simulink model "AMB_NL_2_simulation"  (R2021a)
settings: Solver=ode4  StartTime=0.0  StopTime=ttotal  FixedStep=dtsim  RelTol=1e-3
values from neighbouring files (symbols this model uses):
  a1_b0 = 2.13e13    (= 21300000000000)    [AMB_NL_1_vRTHS_m.m]
  a2 = 4.23e6    (= 4230000)    [AMB_NL_1_vRTHS_m.m]
  a3 = 3.3    [AMB_NL_1_vRTHS_m.m]
  adaptivegain = diag(10.^[8.4 6.2 2.1 0.8])    [AMB_NL_1_vRTHS_m.m]
  Ar = [zeros(3),eye(3);-M\Kmod -M\C]    [AMB_NL_1_vRTHS_m.m]
  asiv = 0.1    [AMB_NL_1_vRTHS_m.m]
  b1 = 425    [AMB_NL_1_vRTHS_m.m]
  b2 = 1e5    (= 100000)    [AMB_NL_1_vRTHS_m.m]
  Br = [zeros(3,2);-ones(3,1),-M\G2]    [AMB_NL_1_vRTHS_m.m]
  ce = 114.6    [AMB_NL_1_vRTHS_m.m]
  Cr = [eye(6)]    [AMB_NL_1_vRTHS_m.m]
  Derivadas = [u;dudt;dudt2;dudt3]    [AMB_NL_1_vRTHS_m.m]
  Dr = [zeros(6,2)]    [AMB_NL_1_vRTHS_m.m]
  dtsim = 1/fs    (= 0.000244140625)    [AMB_NL_1_vRTHS_m.m]
  dudt2 = [1 -2 1 0]/dtsim^2    [AMB_NL_1_vRTHS_m.m]
  gain = 1    [AMB_NL_1_vRTHS_m.m]
  ke = 1.19*10^6    (= 1190000)    [AMB_NL_1_vRTHS_m.m]
  khard = 6e9*0    (= 0)    [AMB_NL_1_vRTHS_m.m]
  max_amb = [amb0max,amb1max,amb2max,amb3max]    [AMB_NL_1_vRTHS_m.m]
  me = 29.1    [AMB_NL_1_vRTHS_m.m]
  min_amb = [amb0min,amb1min,amb2min,amb3min]    [AMB_NL_1_vRTHS_m.m]
  n1siv = 0.1    [AMB_NL_1_vRTHS_m.m]
  n2siv = 1-n1siv    (= 0.9)    [AMB_NL_1_vRTHS_m.m]
  nsiv = 2.5    [AMB_NL_1_vRTHS_m.m]
  rms_noise_desp = 6.25e-14    [AMB_NL_1_vRTHS_m.m]
  rms_noise_F = 1.16e-3    (= 0.00116)    [AMB_NL_1_vRTHS_m.m]
  sat_limit_lower = -3.8    [AMB_NL_1_vRTHS_m.m]
  sat_limit_upper = +3.8    (= 3.8)    [AMB_NL_1_vRTHS_m.m]
  ssAe = [0,1;-asiv*ke/me,-ce/me]    [AMB_NL_1_vRTHS_m.m]
  ssAn = [zeros(3),eye(3);-Mn\Kn,-Mn\Cn]    [AMB_NL_1_vRTHS_m.m]
  ssBe = [0,0;1/me,-1/me]    [AMB_NL_1_vRTHS_m.m]
  ssBn = [zeros(3,2);-Mn\M*G1,-Mn\G2]    [AMB_NL_1_vRTHS_m.m]
  ssCe = [1,0;0,1;asiv*ke,0]    [AMB_NL_1_vRTHS_m.m]
  ssCn = [eye(3),zeros(3)]    [AMB_NL_1_vRTHS_m.m]
  ssDe = [0,0;0,0;0,1]    [AMB_NL_1_vRTHS_m.m]
  ssDn = zeros(3,2)    [AMB_NL_1_vRTHS_m.m]
  stiffdeg = 0.02*0    (= 0)    [AMB_NL_1_vRTHS_m.m]
  strdeg = 0.005*0    (= 0)    [AMB_NL_1_vRTHS_m.m]
  xy = 1/1000    (= 0.001)    [AMB_NL_1_vRTHS_m.m]
undefined symbols (not defined in the file or in its folder): denfilter, DiscIntNeverNeededParam, numfilter
libraries: simulink x2
settings Model: Creator=cristobal  LastModifiedBy=MSI
settings SolverCC: AlgebraicLoopSolver=TrustRegion
settings DataIOCC: ReturnWorkspaceOutputs=off
settings DebuggingCC: SFMachineParentedDataDiag=warning  ArithmeticOperatorsInVariantConditions=warning
settings SFSimCC: SimUseLocalCustomCode=off  CustomCodeUndefinedFunction=UseInterfaceOnly
settings RTWCC: RTWUseLocalCustomCode=off
settings CodeAppCC: StateflowObjectComments=on

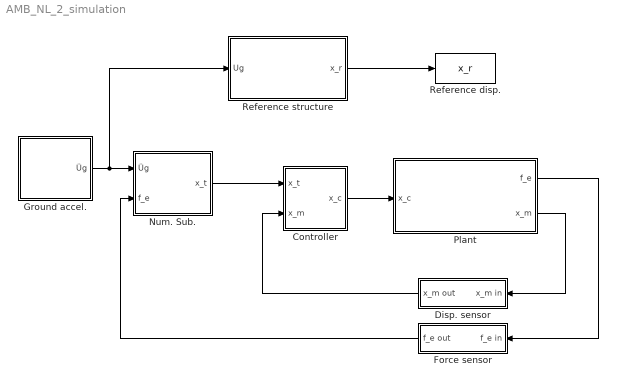
== system AMB_NL_2_simulation ==
  Controller : Subsystem
  Disp. sensor : Subsystem
  Force sensor : Subsystem
  Ground accel. : Subsystem
  Num. Sub. : Subsystem
  Plant : Subsystem
  Reference disp. : ToWorkspace  VariableName=x_r  SaveFormat=Timeseries  SampleTime=-1
  Reference structure : Subsystem
  wires:
  Num. Sub./1(x_t) -> Controller/1(x_t)
  Controller/1(x_c) -> Plant/1(x_c)
  Plant/1(f_e) -> Force sensor/1(f_e in)
  Plant/2(x_m) -> Disp. sensor/1(x_m in)
  Ground accel./1(Üg) -> Num. Sub./1(Üg), Reference structure/1(Ug)
  Reference structure/1(x_r) -> Reference disp./1
  Disp. sensor/1(x_m out) -> Controller/2(x_m)
  Force sensor/1(f_e out) -> Num. Sub./2(f_e)

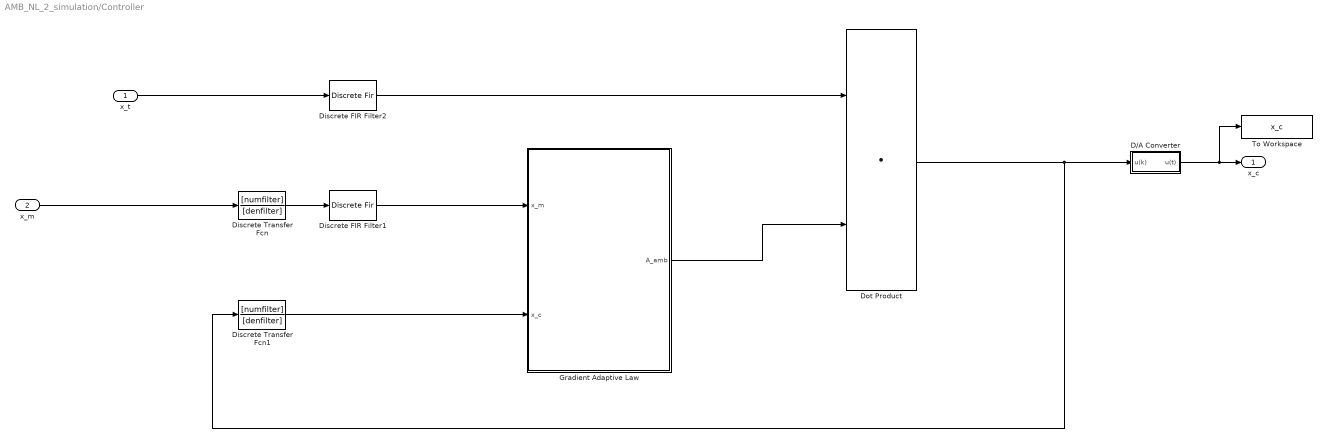
== system AMB_NL_2_simulation/Controller ==
  x_t : Inport
  x_m : Inport  Port=2
  D/A Converter : Subsystem
  Discrete Transfer Fcn : DiscreteTransferFcn  Numerator=[numfilter]  Denominator=[denfilter]
  Discrete Transfer Fcn1 : DiscreteTransferFcn  Numerator=[numfilter]  Denominator=[denfilter]
  Discrete FIR Filter1 : DiscreteFir  Coefficients=Derivadas
  Discrete FIR Filter2 : DiscreteFir  Coefficients=Derivadas
  Dot Product : DotProduct  InputSameDT=on  OutDataTypeStr=Inherit: Inherit via internal rule
  Gradient Adaptive Law : Subsystem
  To Workspace : ToWorkspace  VariableName=x_c  SaveFormat=Timeseries  SampleTime=-1
  x_c : Outport  VectorParamsAs1DForOutWhenUnconnected=off
  wires:
  Gradient Adaptive Law/1(A_amb) -> Dot Product/2
  Discrete FIR Filter1/1 -> Gradient Adaptive Law/1(x_m)
  Discrete Transfer Fcn1/1 -> Gradient Adaptive Law/2(x_c)
  x_m/1 -> Discrete Transfer Fcn/1
  Discrete Transfer Fcn/1 -> Discrete FIR Filter1/1
  x_t/1 -> Discrete FIR Filter2/1
  Dot Product/1 -> D/A Converter/1(u(k)), Discrete Transfer Fcn1/1
  Discrete FIR Filter2/1 -> Dot Product/1
  D/A Converter/1(u(t)) -> To Workspace/1, x_c/1

== system AMB_NL_2_simulation/Disp. sensor ==
  x_m in : Inport
  Band-Limited White Noise : simulink/Sources/Band-Limited White Noise  Cov=[rms_noise_desp]  Ts=dtsim  seed=ceil(rand(1)*10000)
  Sum : Sum  Inputs=|++
  To Workspace : ToWorkspace  VariableName=x_m  SaveFormat=Timeseries  SampleTime=-1
  To Workspace1 : ToWorkspace  VariableName=noise_desp  SaveFormat=Timeseries  SampleTime=-1
  x_m out : Outport  VectorParamsAs1DForOutWhenUnconnected=off
  wires:
  Band-Limited White Noise/1 -> To Workspace1/1, Sum/2
  Sum/1 -> x_m out/1, To Workspace/1
  x_m in/1 -> Sum/1

== system AMB_NL_2_simulation/Force sensor ==
  f_e in : Inport
  Band-Limited White Noise : simulink/Sources/Band-Limited White Noise  Cov=[rms_noise_F]  Ts=dtsim  seed=ceil(rand(1)*100)
  Sum : Sum  Inputs=|++
  To Workspace : ToWorkspace  VariableName=F_m  SaveFormat=Timeseries  SampleTime=-1
  f_e out : Outport  VectorParamsAs1DForOutWhenUnconnected=off
  wires:
  f_e in/1 -> Sum/1
  Sum/1 -> To Workspace/1, f_e out/1
  Band-Limited White Noise/1 -> Sum/2

== system AMB_NL_2_simulation/Ground accel. ==
  From Workspace1 : FromWorkspace  VariableName=Ug  OutputAfterFinalValue=Setting to zero
  To Workspace : ToWorkspace  VariableName=Ugs  SaveFormat=Timeseries  SampleTime=-1
  Üg : Outport  VectorParamsAs1DForOutWhenUnconnected=off
  wires:
  From Workspace1/1 -> To Workspace/1, Üg/1

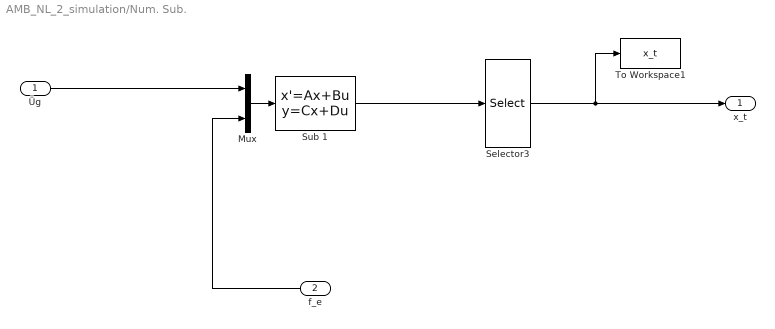
== system AMB_NL_2_simulation/Num. Sub. ==
  Üg : Inport
  f_e : Inport  Port=2
  Mux : Mux  Inputs=2
  Selector3 : Selector  InputPortWidth=3  IndexOptions=Index vector (dialog)  Indices=[1]  OutputSizes=1
  Sub 1 : StateSpace  A=ssAn  B=ssBn  C=ssCn  D=ssDn  InitialCondition=0
  To Workspace1 : ToWorkspace  VariableName=x_t  SaveFormat=Timeseries  SampleTime=-1
  x_t : Outport  VectorParamsAs1DForOutWhenUnconnected=off
  wires:
  Mux/1 -> Sub 1/1
  Selector3/1 -> x_t/1, To Workspace1/1
  Üg/1 -> Mux/1
  Sub 1/1 -> Selector3/1
  f_e/1 -> Mux/2

== system AMB_NL_2_simulation/Plant ==
  x_c : Inport
  Actuator : Subsystem
  Experimental Sub : Subsystem
  f_e : Outport  VectorParamsAs1DForOutWhenUnconnected=off
  x_m : Outport  Port=2  VectorParamsAs1DForOutWhenUnconnected=off
  wires:
  x_c/1 -> Actuator/1(x_c)
  Experimental Sub/2(x_m) -> x_m/1, Actuator/2(x_m)
  Experimental Sub/3(x_m s) -> Actuator/3(x_m s)
  Actuator/1(F) -> Experimental Sub/1(F)
  Experimental Sub/1(F2) -> f_e/1

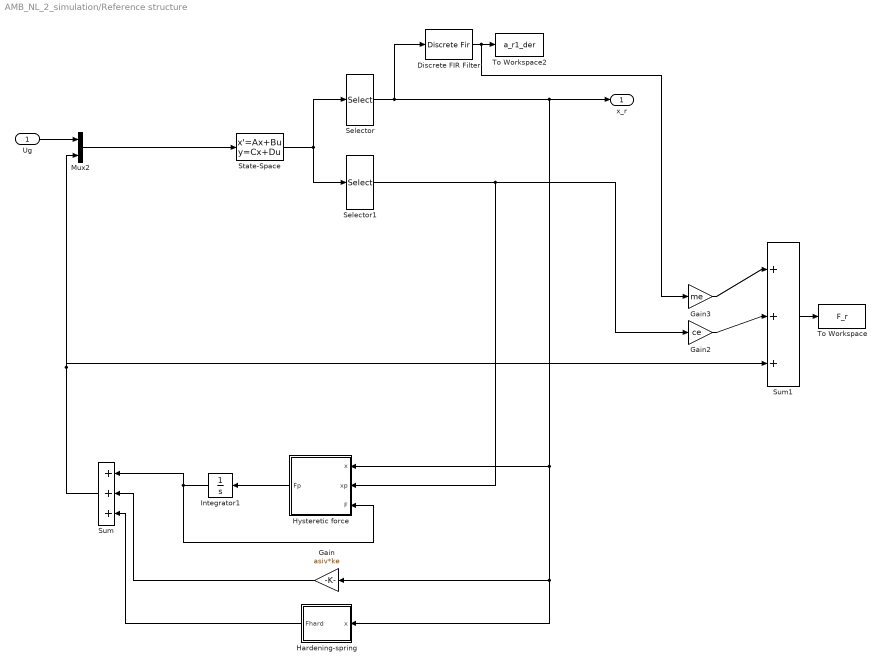
== system AMB_NL_2_simulation/Reference structure ==
  Ug : Inport
  Discrete FIR Filter : DiscreteFir  Coefficients=[dudt2]
  Gain : Gain  Gain=asiv*ke
  Gain2 : Gain  Gain=ce
  Gain3 : Gain  Gain=me
  Hardening-spring : Subsystem
  Hysteretic force : Subsystem
  Integrator1 : Integrator
  Mux2 : Mux  Inputs=2
  Selector : Selector  InputPortWidth=6  IndexOptions=Index vector (dialog)  Indices=[1]  OutputSizes=1
  Selector1 : Selector  InputPortWidth=6  IndexOptions=Index vector (dialog)  Indices=[4]  OutputSizes=1
  State-Space : StateSpace  A=Ar  B=Br  C=Cr  D=Dr  InitialCondition=0
  Sum : Sum  Inputs=|+++
  Sum1 : Sum  Inputs=|+++
  To Workspace : ToWorkspace  VariableName=F_r  SaveFormat=Timeseries  SampleTime=-1
  To Workspace2 : ToWorkspace  VariableName=a_r1_der  SaveFormat=Timeseries  SampleTime=-1
  x_r : Outport  VectorParamsAs1DForOutWhenUnconnected=off
  wires:
  State-Space/1 -> Selector1/1, Selector/1
  Selector/1 -> Discrete FIR Filter/1, Hardening-spring/1(x), Gain/1, Hysteretic force/1(x), x_r/1
  Selector1/1 -> Hysteretic force/2(xp), Gain2/1
  Mux2/1 -> State-Space/1
  Ug/1 -> Mux2/1
  Integrator1/1 -> Hysteretic force/3(F), Sum/1
  Gain/1 -> Sum/2
  Sum1/1 -> To Workspace/1
  Discrete FIR Filter/1 -> Gain3/1, To Workspace2/1
  Gain2/1 -> Sum1/2
  Gain3/1 -> Sum1/1
  Hysteretic force/1(Fp) -> Integrator1/1
  Sum/1 -> Mux2/2, Sum1/3
  Hardening-spring/1(Fhard) -> Sum/3

== system AMB_NL_2_simulation/Controller/D//A Converter ==
  u(k) : Inport
  Quantizer : Quantizer  QuantizationInterval=quantize_int
  Saturation : Saturate  UpperLimit=sat_limit_upper  LowerLimit=sat_limit_lower
  u(t) : Outport  VectorParamsAs1DForOutWhenUnconnected=off
  wires:
  Saturation/1 -> u(t)/1
  Quantizer/1 -> Saturation/1
  u(k)/1 -> Quantizer/1

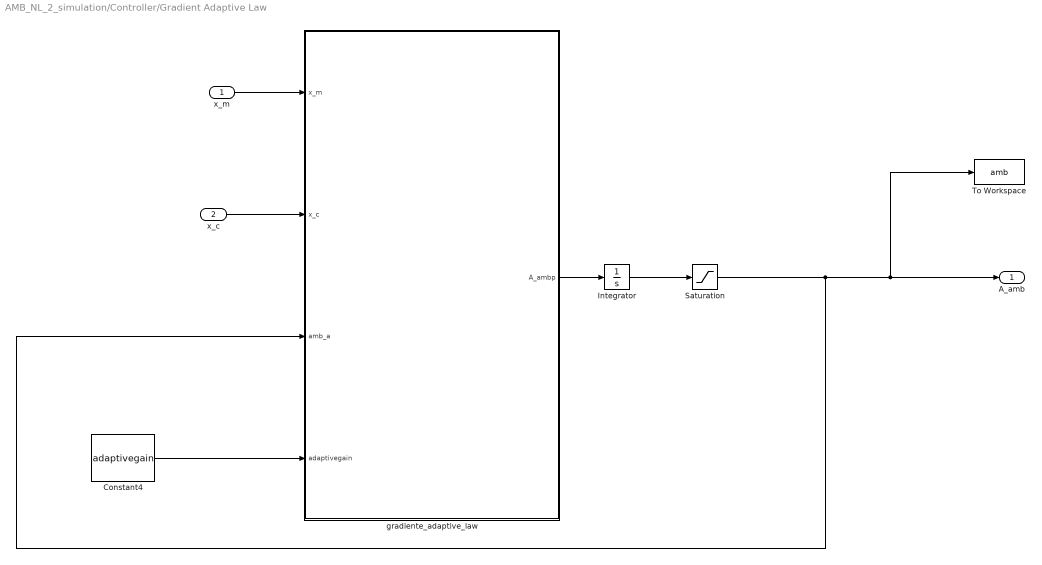
== system AMB_NL_2_simulation/Controller/Gradient Adaptive Law ==
  x_m : Inport
  x_c : Inport  Port=2
  Constant4 : Constant  Value=adaptivegain
  Integrator : Integrator  InitialCondition=A_amb_i'
  Saturation : Saturate  UpperLimit=[max_amb]  LowerLimit=min_amb
  To Workspace : ToWorkspace  VariableName=amb  SaveFormat=Timeseries  SampleTime=-1
  gradiente_adaptive_law : MATLAB Function  TreatAsAtomicUnit=on
  A_amb : Outport  VectorParamsAs1DForOutWhenUnconnected=off
  wires:
  Saturation/1 -> gradiente_adaptive_law/3(amb_a), To Workspace/1, A_amb/1
  Integrator/1 -> Saturation/1
  x_c/1 -> gradiente_adaptive_law/2(x_c)
  Constant4/1 -> gradiente_adaptive_law/4(adaptivegain)
  gradiente_adaptive_law/1(A_ambp) -> Integrator/1
  x_m/1 -> gradiente_adaptive_law/1(x_m)

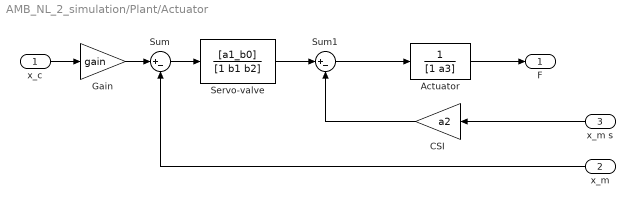
== system AMB_NL_2_simulation/Plant/Actuator ==
  x_c : Inport
  x_m : Inport  Port=2
  x_m s : Inport  Port=3
  Actuator : TransferFcn  Denominator=[1 a3]
  CSI : Gain  Gain=a2
  Gain : Gain  Gain=gain
  Servo-valve : TransferFcn  Numerator=[a1_b0]  Denominator=[1 b1 b2]
  Sum : Sum  Inputs=|+-
  Sum1 : Sum  Inputs=|+-
  F : Outport  VectorParamsAs1DForOutWhenUnconnected=off
  wires:
  CSI/1 -> Sum1/2
  Actuator/1 -> F/1
  Sum1/1 -> Actuator/1
  Sum/1 -> Servo-valve/1
  Servo-valve/1 -> Sum1/1
  x_c/1 -> Gain/1
  Gain/1 -> Sum/1
  x_m/1 -> Sum/2
  x_m s/1 -> CSI/1

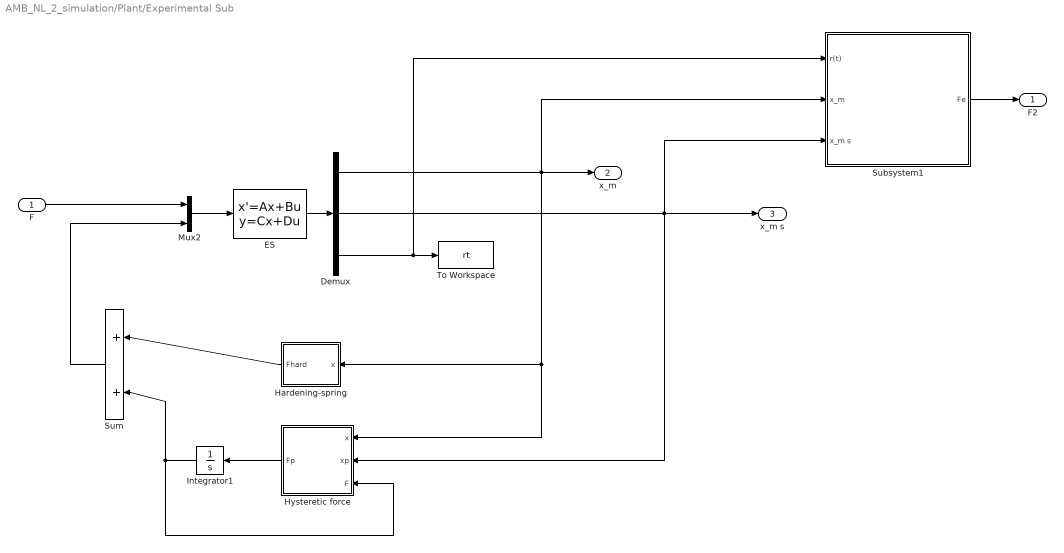
== system AMB_NL_2_simulation/Plant/Experimental Sub ==
  F : Inport
  Demux : Demux  Outputs=3
  ES : StateSpace  A=ssAe  B=ssBe  C=ssCe  D=ssDe  InitialCondition=0
  Hardening-spring : Subsystem
  Hysteretic force : Subsystem
  Integrator1 : Integrator
  Mux2 : Mux  Inputs=2
  Subsystem1 : Subsystem
  Sum : Sum  Inputs=|++
  To Workspace : ToWorkspace  VariableName=rt  SaveFormat=Timeseries  SampleTime=-1
  F2 : Outport  VectorParamsAs1DForOutWhenUnconnected=off
  x_m : Outport  Port=2  VectorParamsAs1DForOutWhenUnconnected=off
  x_m s : Outport  Port=3  VectorParamsAs1DForOutWhenUnconnected=off
  wires:
  ES/1 -> Demux/1
  F/1 -> Mux2/1
  Mux2/1 -> ES/1
  Demux/3 -> Subsystem1/1(r(t)), To Workspace/1
  Hysteretic force/1(Fp) -> Integrator1/1
  Demux/2 -> Hysteretic force/2(xp), Subsystem1/3(x_m s), x_m s/1
  Subsystem1/1(Fe) -> F2/1
  Demux/1 -> x_m/1, Hysteretic force/1(x), Hardening-spring/1(x), Subsystem1/2(x_m)
  Integrator1/1 -> Sum/2, Hysteretic force/3(F)
  Sum/1 -> Mux2/2
  Hardening-spring/1(Fhard) -> Sum/1

== system AMB_NL_2_simulation/Reference structure/Hardening-spring ==
  x : Inport
  Constant1 : Constant  Value=khard
  MATLAB Function : MATLAB Function  TreatAsAtomicUnit=on
  Unit Delay : UnitDelay  SampleTime=-1  HasFrameUpgradeWarning=on
  Fhard : Outport  VectorParamsAs1DForOutWhenUnconnected=off
  wires:
  x/1 -> Unit Delay/1
  Constant1/1 -> MATLAB Function/2(khard)
  MATLAB Function/1(Fhard) -> Fhard/1
  Unit Delay/1 -> MATLAB Function/1(x)

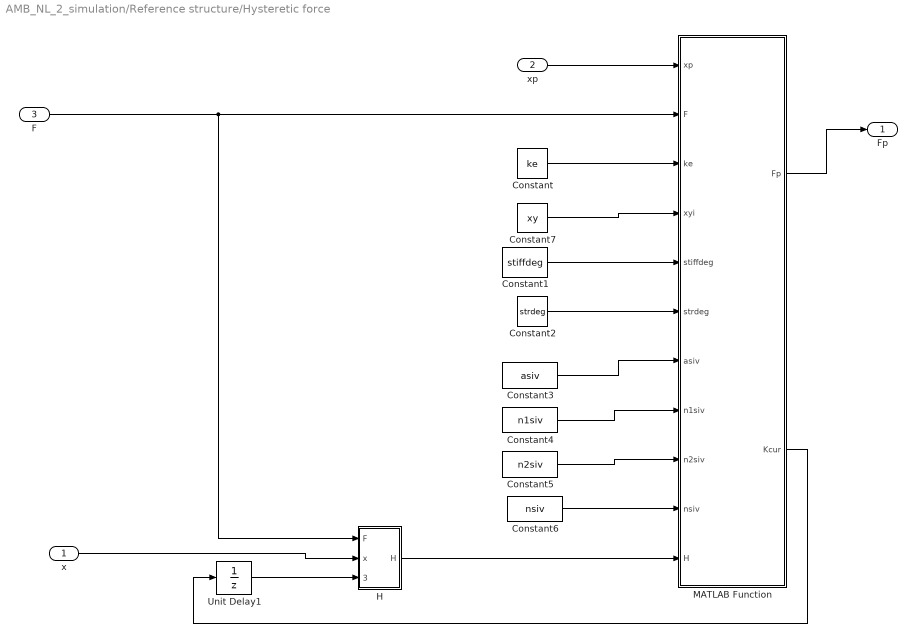
== system AMB_NL_2_simulation/Reference structure/Hysteretic force ==
  x : Inport
  xp : Inport  Port=2
  F : Inport  Port=3
  Constant : Constant  Value=ke
  Constant1 : Constant  Value=stiffdeg
  Constant2 : Constant  Value=strdeg
  Constant3 : Constant  Value=asiv
  Constant4 : Constant  Value=n1siv
  Constant5 : Constant  Value=n2siv
  Constant6 : Constant  Value=nsiv
  Constant7 : Constant  Value=xy
  H : Subsystem
  MATLAB Function : MATLAB Function  TreatAsAtomicUnit=on
  Unit Delay1 : UnitDelay  InitialCondition=ke  SampleTime=-1  HasFrameUpgradeWarning=on
  Fp : Outport  VectorParamsAs1DForOutWhenUnconnected=off
  wires:
  MATLAB Function/1(Fp) -> Fp/1
  MATLAB Function/2(Kcur) -> Unit Delay1/1
  x/1 -> H/2(x)
  xp/1 -> MATLAB Function/1(xp)
  Constant/1 -> MATLAB Function/3(ke)
  Constant7/1 -> MATLAB Function/4(xyi)
  Constant1/1 -> MATLAB Function/5(stiffdeg)
  Constant2/1 -> MATLAB Function/6(strdeg)
  Constant3/1 -> MATLAB Function/7(asiv)
  Constant4/1 -> MATLAB Function/8(n1siv)
  Constant5/1 -> MATLAB Function/9(n2siv)
  Constant6/1 -> MATLAB Function/10(nsiv)
  H/1(H) -> MATLAB Function/11(H)
  Unit Delay1/1 -> H/3("Kcur ")
  F/1 -> H/1(F), MATLAB Function/2(F)

== system AMB_NL_2_simulation/Plant/Experimental Sub/Hardening-spring ==
  x : Inport
  Constant1 : Constant  Value=khard
  MATLAB Function : MATLAB Function  TreatAsAtomicUnit=on
  Unit Delay : UnitDelay  SampleTime=-1  HasFrameUpgradeWarning=on
  Fhard : Outport  VectorParamsAs1DForOutWhenUnconnected=off
  wires:
  x/1 -> Unit Delay/1
  Constant1/1 -> MATLAB Function/2(khard)
  MATLAB Function/1(Fhard) -> Fhard/1
  Unit Delay/1 -> MATLAB Function/1(x)

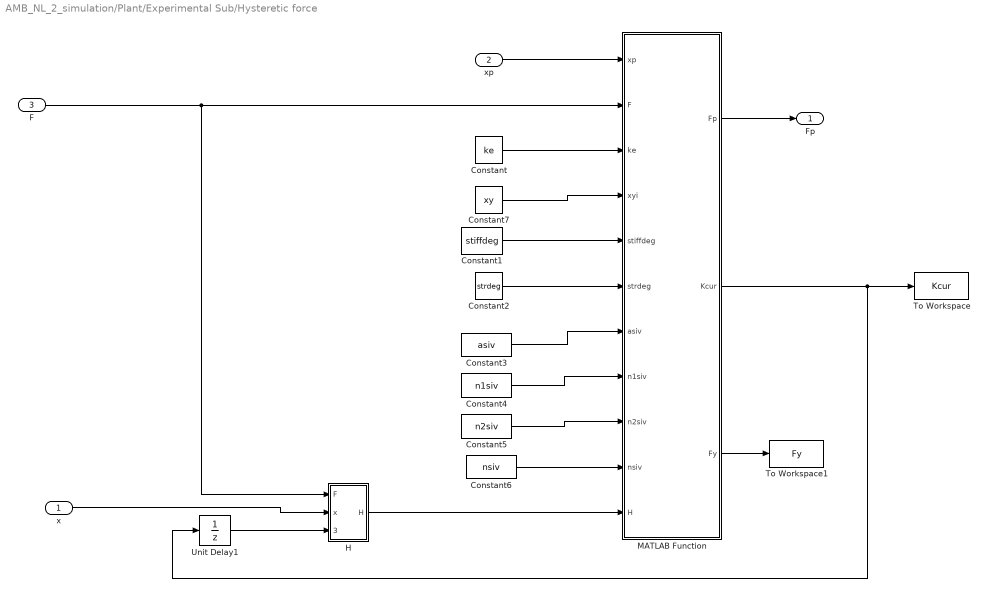
== system AMB_NL_2_simulation/Plant/Experimental Sub/Hysteretic force ==
  x : Inport
  xp : Inport  Port=2
  F : Inport  Port=3
  Constant : Constant  Value=ke
  Constant1 : Constant  Value=stiffdeg
  Constant2 : Constant  Value=strdeg
  Constant3 : Constant  Value=asiv
  Constant4 : Constant  Value=n1siv
  Constant5 : Constant  Value=n2siv
  Constant6 : Constant  Value=nsiv
  Constant7 : Constant  Value=xy
  H : Subsystem
  MATLAB Function : MATLAB Function  TreatAsAtomicUnit=on
  To Workspace : ToWorkspace  VariableName=Kcur  SaveFormat=Timeseries  SampleTime=-1
  To Workspace1 : ToWorkspace  VariableName=Fy  SaveFormat=Timeseries  SampleTime=-1
  Unit Delay1 : UnitDelay  InitialCondition=ke  SampleTime=-1  HasFrameUpgradeWarning=on
  Fp : Outport  VectorParamsAs1DForOutWhenUnconnected=off
  wires:
  MATLAB Function/1(Fp) -> Fp/1
  MATLAB Function/2(Kcur) -> Unit Delay1/1, To Workspace/1
  x/1 -> H/2(x)
  xp/1 -> MATLAB Function/1(xp)
  Constant/1 -> MATLAB Function/3(ke)
  Constant7/1 -> MATLAB Function/4(xyi)
  Constant1/1 -> MATLAB Function/5(stiffdeg)
  Constant2/1 -> MATLAB Function/6(strdeg)
  Constant3/1 -> MATLAB Function/7(asiv)
  Constant4/1 -> MATLAB Function/8(n1siv)
  Constant5/1 -> MATLAB Function/9(n2siv)
  Constant6/1 -> MATLAB Function/10(nsiv)
  H/1(H) -> MATLAB Function/11(H)
  Unit Delay1/1 -> H/3("Kcur ")
  F/1 -> H/1(F), MATLAB Function/2(F)
  MATLAB Function/3(Fy) -> To Workspace1/1

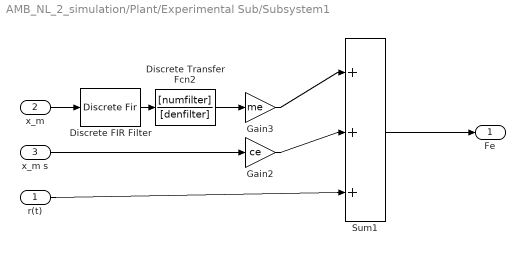
== system AMB_NL_2_simulation/Plant/Experimental Sub/Subsystem1 ==
  r(t) : Inport
  x_m : Inport  Port=2
  x_m s : Inport  Port=3
  Discrete Transfer Fcn2 : DiscreteTransferFcn  Numerator=[numfilter]  Denominator=[denfilter]
  Discrete FIR Filter : DiscreteFir  Coefficients=[dudt2]
  Gain2 : Gain  Gain=ce
  Gain3 : Gain  Gain=me
  Sum1 : Sum  Inputs=|+++
  Fe : Outport  VectorParamsAs1DForOutWhenUnconnected=off
  wires:
  Sum1/1 -> Fe/1
  Discrete FIR Filter/1 -> Discrete Transfer Fcn2/1
  Discrete Transfer Fcn2/1 -> Gain3/1
  Gain3/1 -> Sum1/1
  Gain2/1 -> Sum1/2
  r(t)/1 -> Sum1/3
  x_m s/1 -> Gain2/1
  x_m/1 -> Discrete FIR Filter/1

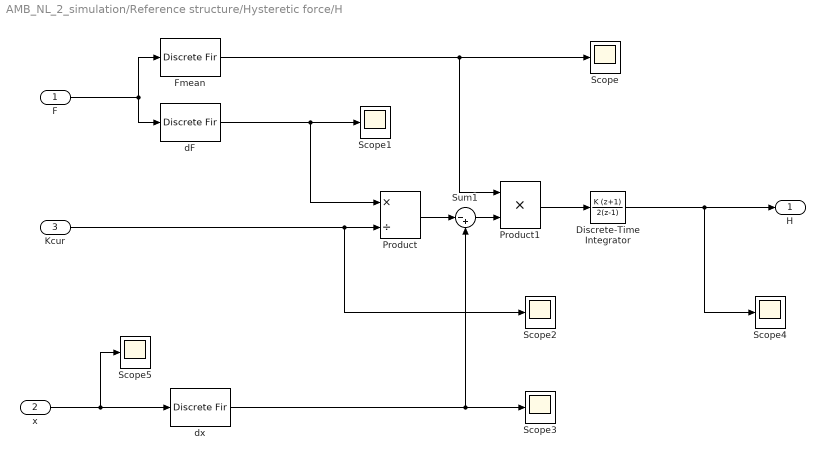
== system AMB_NL_2_simulation/Reference structure/Hysteretic force/H ==
  F : Inport
  x : Inport  Port=2
  "Kcur " : Inport  Port=3
  Discrete-Time Integrator : DiscreteIntegrator  IntegratorMethod=Accumulation: Trapezoidal  SampleTime=-1  ICPrevOutput=DiscIntNeverNeededParam  ICPrevScaledInput=DiscIntNeverNeededParam
  Fmean : DiscreteFir
  Product : Product  Inputs=*/
  Product1 : Product
  Scope{,1..5} (6 alike) : Scope
  Sum1 : Sum  Inputs=|-+
  dF : DiscreteFir  Coefficients=[1 -1]
  dx : DiscreteFir  Coefficients=[1 -1]
  H : Outport  VectorParamsAs1DForOutWhenUnconnected=off
  wires:
  dF/1 -> Scope1/1, Product/1
  "Kcur "/1 -> Scope2/1, Product/2
  Product1/1 -> Discrete-Time Integrator/1
  Sum1/1 -> Product1/2
  x/1 -> Scope5/1, dx/1
  F/1 -> Fmean/1, dF/1
  Discrete-Time Integrator/1 -> Scope4/1, H/1
  Product/1 -> Sum1/1
  dx/1 -> Scope3/1, Sum1/2
  Fmean/1 -> Scope/1, Product1/1

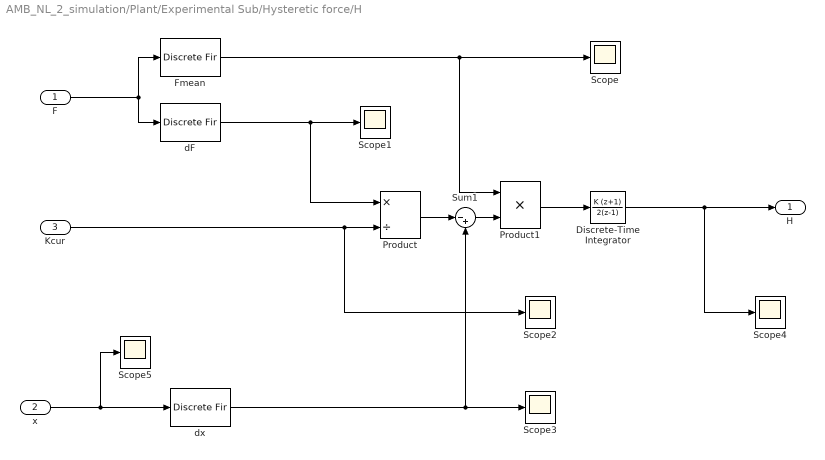
== system AMB_NL_2_simulation/Plant/Experimental Sub/Hysteretic force/H ==
  F : Inport
  x : Inport  Port=2
  "Kcur " : Inport  Port=3
  Discrete-Time Integrator : DiscreteIntegrator  IntegratorMethod=Accumulation: Trapezoidal  SampleTime=-1  ICPrevOutput=DiscIntNeverNeededParam  ICPrevScaledInput=DiscIntNeverNeededParam
  Fmean : DiscreteFir
  Product : Product  Inputs=*/
  Product1 : Product
  Scope{,1..5} (6 alike) : Scope
  Sum1 : Sum  Inputs=|-+
  dF : DiscreteFir  Coefficients=[1 -1]
  dx : DiscreteFir  Coefficients=[1 -1]
  H : Outport  VectorParamsAs1DForOutWhenUnconnected=off
  wires:
  dF/1 -> Scope1/1, Product/1
  "Kcur "/1 -> Scope2/1, Product/2
  Product1/1 -> Discrete-Time Integrator/1
  Sum1/1 -> Product1/2
  x/1 -> Scope5/1, dx/1
  F/1 -> Fmean/1, dF/1
  Discrete-Time Integrator/1 -> Scope4/1, H/1
  Product/1 -> Sum1/1
  dx/1 -> Scope3/1, Sum1/2
  Fmean/1 -> Scope/1, Product1/1

== matlab function AMB_NL_2_simulation/Reference structure/Hysteretic force/MATLAB Function ==
  data: xp input; F input; Fp output; ke input; xyi input; stiffdeg input; strdeg input; asiv input; n1siv input; n2siv input; nsiv input; Kcur output; H input
function [Fp,Kcur] = stiffdegradation(xp,F,ke,xyi,stiffdeg,strdeg,asiv,n1siv,n2siv,nsiv,H)
%stiffnes degradation
Kcur=((exp(-stiffdeg*H))-asiv)*ke; %(((1+stiffdeg*H)^-1)-asiv)*ke;
%Max displacement
%Yield force
Fyi=(1-asiv)*ke*xyi;
Fy=Fyi*(1+strdeg*H)^-1;
if Fy<=0.01*Fyi
    Fy=Fyi*0.01;
end
%current stiffness
Khyst=Kcur*(1-abs(F/Fy)^(nsiv)*(n1siv*sign(F*xp)+n2siv));

Fp=Khyst*xp;

== matlab function AMB_NL_2_simulation/Controller/Gradient Adaptive Law/gradiente_adaptive_law ==
  data: x_m input; x_c input; amb_a input; A_ambp output; adaptivegain input
function A_ambp   = fcn(x_m,x_c,amb_a,adaptivegain)
error=(x_c-amb_a'*x_m)/(1+(x_m'*x_m));
A_ambp=adaptivegain*error*x_m;

== matlab function AMB_NL_2_simulation/Plant/Experimental Sub/Hysteretic force/MATLAB Function ==
  data: xp input; F input; Fp output; ke input; xyi input; stiffdeg input; strdeg input; asiv input; n1siv input; n2siv input; nsiv input; Kcur output; H input; Fy output
function [Fp,Kcur,Fy] = stiffdegradation(xp,F,ke,xyi,stiffdeg,strdeg,asiv,n1siv,n2siv,nsiv,H)
%stiffnes degradation
Kcur=((exp(-stiffdeg*H))-asiv)*ke; %(((1+stiffdeg*H)^-1)-asiv)*ke;
%Max displacement
%Yield force
Fyi=(1-asiv)*ke*xyi;
Fy=Fyi*(1+strdeg*H)^-1;
if Fy<=0.01*Fyi
    Fy=Fyi*0.01;
end
%current stiffness
Khyst=Kcur*(1-abs(F/Fy)^(nsiv)*(n1siv*sign(F*xp)+n2siv));

Fp=Khyst*xp;

== matlab function AMB_NL_2_simulation/Plant/Experimental Sub/Hardening-spring/MATLAB Function ==
  data: x input; Fhard output; khard input
function Fhard  = hardening(x,khard)
Fhard=khard*(x^3);

== matlab function AMB_NL_2_simulation/Reference structure/Hardening-spring/MATLAB Function ==
  data: x input; Fhard output; khard input
function Fhard  = hardening(x,khard)
Fhard=khard*(x^3);
